simulink library "lwdf_adaptors"  (R2014b)
settings: Solver=ode45  StartTime=0.0  StopTime=10.0  RelTol=1e-3
settings Model: Creator=ravoson  LastModifiedBy=ravoson

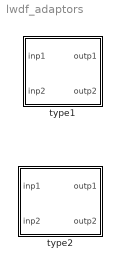
== system lwdf_adaptors ==
  type1 : Subsystem
  type2 : Subsystem

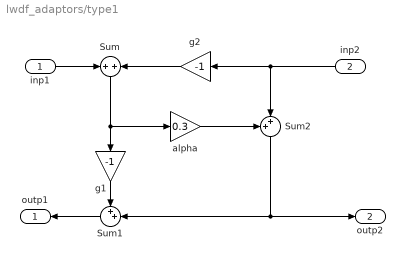
== system lwdf_adaptors/type1 ==
  inp1 : Inport
  inp2 : Inport  Port=2
  Sum : Sum  Inputs=+|+
  Sum1 : Sum  Inputs=++|
  Sum2 : Sum  Inputs=++|
  alpha : Gain  Gain=0.3
  g1 : Gain  Gain=-1
  g2 : Gain  Gain=-1
  outp1 : Outport
  outp2 : Outport  Port=2
  wires:
  alpha/1 -> Sum2/1
  Sum/1 -> alpha/1, g1/1
  g1/1 -> Sum1/1
  inp1/1 -> Sum/1
  Sum2/1 -> outp2/1, Sum1/2
  inp2/1 -> Sum2/2, g2/1
  Sum1/1 -> outp1/1
  g2/1 -> Sum/2

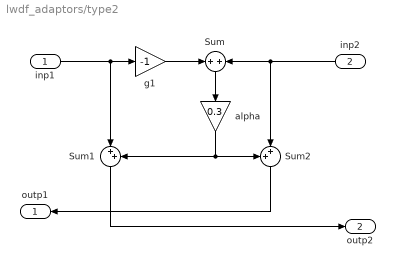
== system lwdf_adaptors/type2 ==
  inp1 : Inport
  inp2 : Inport  Port=2
  Sum : Sum  Inputs=+|+
  Sum1 : Sum  Inputs=|++
  Sum2 : Sum  Inputs=++|
  alpha : Gain  Gain=0.3
  g1 : Gain  Gain=-1
  outp1 : Outport
  outp2 : Outport  Port=2
  wires:
  alpha/1 -> Sum1/2, Sum2/1
  Sum/1 -> alpha/1
  Sum1/1 -> outp2/1
  inp2/1 -> Sum2/2, Sum/2
  g1/1 -> Sum/1
  Sum2/1 -> outp1/1
  inp1/1 -> Sum1/1, g1/1
